simulink model "kalman_vision"  (R2013a)
settings: Solver=ode3  StartTime=0.0  StopTime=Inf  FixedStep=1/30  RelTol=1e-3
undefined symbols (not defined in the file or in its folder): none, serial, strel, videoinput
libraries: visionsinks x3, instrumentlib x3, simulink x2, visionstatistics x1, imaqlib x1, visiontextngfix x1, dspadpt3 x1, visionmorphops x1
settings Model: Creator=Michael  LastModifiedBy=nano

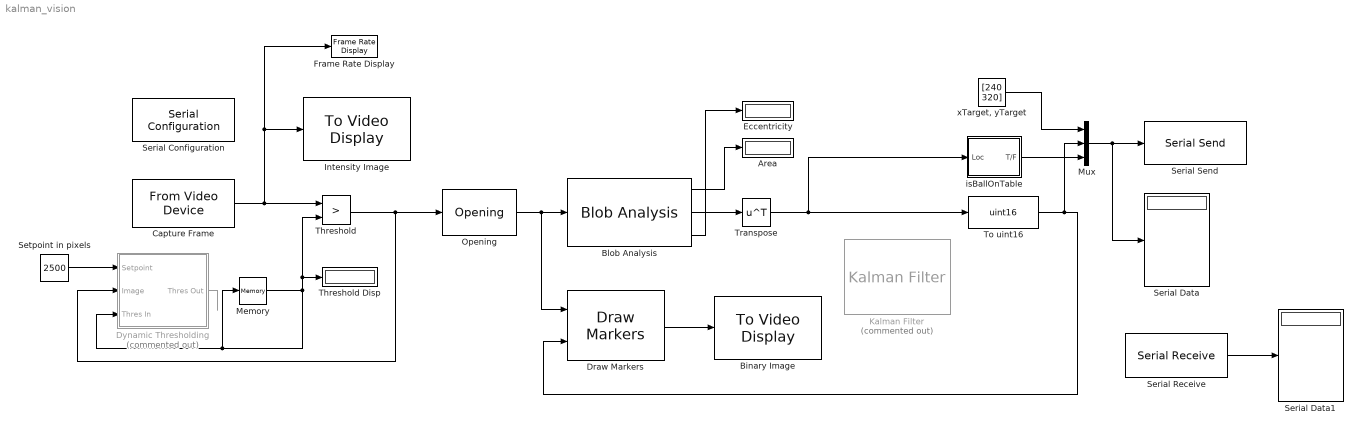
== system kalman_vision ==
  Area : Display
  Binary Image : visionsinks/To Video Display  inputType=Obsolete  imagePorts=One multidimensional signal  OutputDevice=On-screen video monitor  fullScreen=off  videoWindowX=-732  videoWindowY=343  saveWindowSize=off  videoWindowWidth=640  videoWindowHeight=480  dataOrg=Column-major  openAtMdlStart=on  isWindowOpen=off  inputColorFormat=RGB
  Blob Analysis : visionstatistics/Blob Analysis  Tag=vipblks_row_conv  area=on  centroid=on  bBox=off  majorAxis=off  minorAxis=off  angle=off  eccentricity=on  equivDiameterSq=off  extent=off  perimeter=off  maxBlobs=1  warnIfNumBlobsExceeded=off  isCount=off  useMinArea=on  minArea=700  useMaxArea=on  maxArea=2000  excludeBorderBlob=on  outDT=double  isOutVarDim=off  isFill=on  fillValues=-1  conn=8  isLabel=off  outputMode=Binary point scaling  outputWordLength=32  outputFracLength=16  firstCoeffMode=Binary point scaling  firstCoeffWordLength=16  firstCoeffFracLength=14  secondCoeffMode=Binary point scaling  secondCoeffWordLength=32  secondCoeffFracLength=16  accumMode=Binary point scaling  accumWordLength=32  accumFracLength=0  prodOutputMode=Binary point scaling  prodOutputWordLength=32  prodOutputFracLength=16  roundingMode=Floor  overflowMode=off
  Capture Frame : imaqlib/From Video Device  DeviceMenu=winvideo 1 (HP Prem AF Webcam KQ245AA)  Device=winvideo 1 (HP Prem AF Webcam KQ245AA)  ObjConstructor=videoinput('winvideo', 1)  VideoFormatMenu=MJPG_640x480  VideoFormat=MJPG_640x480  VideoSource=input1  ROIPosition=[0 0 480 640]  EnableHWTrigger=off  TriggerConfiguration=none/none  SampleTime=1/30  OutputPortsMode=One multidimensional signal  DataType=uint8  CanDoHWTrigger=no  ReturnedColorSpace=grayscale  BlockHandle=1913.0001  ROIWidth=640  ROIHeight=480  ROIColumn=0  ROIRow=0  EngXMLPath=C:\Program Files\MATLAB\R2013a\toolbox\imaq\imaq\private  DevXMLPath=C:\Program Files\MATLAB\R2013a\toolbox\imaq\imaqadaptors\win64  EngLibPath=C:\Program Files\MATLAB\R2013a\toolbox\imaq\imaqblks\imaqmex\win64  ColorSpace=grayscale  BayerSensorAlignment=grbg
  Draw Markers : visiontextngfix/Draw Markers  shape=Plus  size=40  fill=off  fillClrSource=Specify via dialog  display=White  intensity=200  color=[255 0 0]  opacity=0.6  viewport=Entire image  antialiasing=off  inType=Obsolete  imagePorts=One multidimensional signal  prodOutputMode=Binary point scaling  prodOutputWordLength=32  prodOutputFracLength=14  memoryMode=Specify word length  memoryWordLength=16  memoryFracLength=15  roundingMode=Floor  overflowMode=off
  Dynamic Thresholding : Subsystem  Commented=on
  Eccentricity : Display
  Frame Rate Display : visionsinks/Frame Rate Display  UpdateRate=30
  Intensity Image : visionsinks/To Video Display  inputType=Obsolete  imagePorts=One multidimensional signal  OutputDevice=On-screen video monitor  fullScreen=off  videoWindowX=-1279  videoWindowY=60  saveWindowSize=off  videoWindowWidth=640  videoWindowHeight=480  dataOrg=Column-major  openAtMdlStart=on  isWindowOpen=off  inputColorFormat=RGB
  Kalman Filter : dspadpt3/Kalman Filter  Commented=on  num_targets=1  sourceEnable=Always  isReset=on  X=[1; 1; 0; 0; 0; 0]  P=0.5*eye(6)  A=[1 0 1/30 0 (1/30^2)/2 0; 0 1 0 1/30 0 (1/30^2)/2; 0 0 1 0 1/30 0; 0 0 0 1 0 1/30; 0 0 0 0 1 0; 0 0 0 0 0 1]  sourceMeasure=Specify via Dialog  H=[1 0 0 0 0 0; 0 1 0 0 0 0]  Q=diag([(1/30^4)/4 (1/30^4)/4 (1/30)^2 (1/30)^2 1 1])  R=eye(2)  isOutputEstMeasure=on  isOutputEstState=off  isOutputEstError=off  isOutputPrdMeasure=off  isOutputPrdState=off  isOutputPrdError=off
  Memory : Memory  X0=200  InheritSampleTime=on
  Mux : Mux  Inputs=3
  Opening : visionmorphops/Opening  nhoodsrc=Specify via dialog  strel=strel('disk',7)
  Serial Configuration : instrumentlib/Serial Configuration  Priority=-200000  ComPortMenu=COM7  ComPort=COM7  ObjConstructor=serial('COM7');  BaudRate=115200  DataBits=8  Parity=none  StopBits=1  FlowControl=none  Timeout=10  ByteOrder=LittleEndian
  Serial Data : Display
  Serial Data1 : Display
  Serial Receive : instrumentlib/Serial Receive  ComPortMenu=COM7  ComPort=COM7  ObjConstructor=serial('COM7');  Terminator=<none>  DataSize="[5  1]"  DataType=uint16  EnableBlockingMode=on  ActionDataUnavailable=Output custom value  CustomValue=0  SampleTime=1/30
  Serial Send : instrumentlib/Serial Send  ComPortMenu=COM7  ComPort=COM7  ObjConstructor=serial('COM7');  Terminator=<none>  EnableBlockingMode=off
  Setpoint in pixels : Constant  Value=2500  OutDataTypeStr=uint16
  Threshold : RelationalOperator  Operator=>  OutDataTypeStr=boolean  ZeroCross=off
  Threshold Disp : Display
  To uint16 : DataTypeConversion  OutDataTypeStr=uint16
  Transpose : Math  Operator=transpose  SaturateOnIntegerOverflow=on
  isBallOnTable : Subsystem
  "xTarget, yTarget" : Constant  Value=[240 320]  OutDataTypeStr=uint16
  wires:
  Capture Frame/1 -> Frame Rate Display/1, Intensity Image/1, Threshold/1
  To uint16/1 -> Mux/2, Draw Markers/2
  Blob Analysis/1 -> Area/1
  Opening/1 -> Draw Markers/1, Blob Analysis/1
  Draw Markers/1 -> Binary Image/1
  Blob Analysis/3 -> Eccentricity/1
  Blob Analysis/2 -> Transpose/1
  Transpose/1 -> isBallOnTable/1(Loc), To uint16/1
  Mux/1 -> Serial Send/1, Serial Data/1
  "xTarget, yTarget"/1 -> Mux/1
  isBallOnTable/1(T/F) -> Mux/3
  Threshold/1 -> Dynamic Thresholding/2(Image), Opening/1
  Dynamic Thresholding/1(Thres Out) -> ?
  Setpoint in pixels/1 -> Dynamic Thresholding/1(Setpoint)
  Memory/1 -> Threshold/2, Threshold Disp/1, Memory/1, Dynamic Thresholding/3(Thres In)
  Serial Receive/1 -> Serial Data1/1

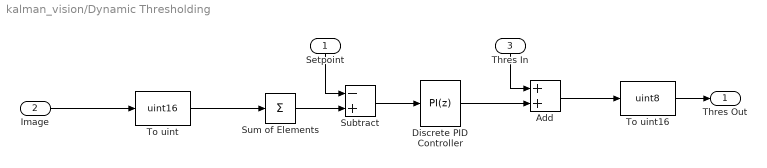
== system kalman_vision/Dynamic Thresholding ==
  Setpoint : Inport
  Image : Inport  Port=2
  Thres In : Inport  Port=3
  Add : Sum
  Discrete PID Controller : simulink/Continuous/PID Controller  Controller=PI  TimeDomain=Discrete-time  SampleTime=-1  IntegratorMethod=Forward Euler  FilterMethod=Forward Euler  Form=Parallel  P=1/5000  I=1/5000  D=0  N=100  InitialConditionSource=internal  InitialConditionForIntegrator=0  InitialConditionForFilter=0  ExternalReset=none  LimitOutput=off  UpperSaturationLimit=50  LowerSaturationLimit=-50  LinearizeAsGain=off  AntiWindupMode=none  Kb=1  TrackingMode=off  Kt=1  PParamMin=[]  PParamMax=[]  IParamMin=[]  IParamMax=[]  DParamMin=[]  DParamMax=[]  NParamMin=[]  NParamMax=[]  KbParamMin=[]  KbParamMax=[]  KtParamMin=[]  KtParamMax=[]  POutMin=[]  POutMax=[]  IOutMin=[]  IOutMax=[]  DOutMin=[]  DOutMax=[]  NOutMin=[]  NOutMax=[]  KbOutMin=[]  KbOutMax=[]  KtOutMin=[]  KtOutMax=[]  IntegratorOutMin=[]  IntegratorOutMax=[]  FilterOutMin=[]  FilterOutMax=[]  SumOutMin=[]  SumOutMax=[]  SumI1OutMin=[]  SumI1OutMax=[]  SumI2OutMin=[]  SumI2OutMax=[]  SumI3OutMin=[]  SumI3OutMax=[]  SumDOutMin=[]  SumDOutMax=[]  SaturationOutMin=[]  SaturationOutMax=[]  IntegratorContinuousStateAttributes=''  IntegratorStateMustResolveToSignalObject=off  IntegratorRTWStateStorageClass=Auto  FilterContinuousStateAttributes=''  FilterStateMustResolveToSignalObject=off  FilterRTWStateStorageClass=Auto
  Subtract : Sum  Inputs=-+  AccumDataTypeStr=single
  Sum of Elements : Sum  Inputs=+
  To uint : DataTypeConversion  OutDataTypeStr=uint16
  To uint16 : DataTypeConversion  OutDataTypeStr=uint8
  Thres Out : Outport
  wires:
  Sum of Elements/1 -> Subtract/2
  Discrete PID Controller/1 -> Add/2
  Subtract/1 -> Discrete PID Controller/1
  Setpoint/1 -> Subtract/1
  Add/1 -> To uint16/1
  Thres In/1 -> Add/1
  Image/1 -> To uint/1
  To uint/1 -> Sum of Elements/1
  To uint16/1 -> Thres Out/1

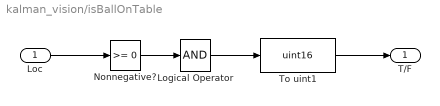
== system kalman_vision/isBallOnTable ==
  Loc : Inport
  Logical Operator : Logic  Inputs=1  AllPortsSameDT=off  OutDataTypeStr=boolean
  Nonnegative? : simulink/Logic and Bit Operations/Compare To Zero  relop=>=  OutDataTypeStr=boolean  ZeroCross=off
  To uint1 : DataTypeConversion  OutDataTypeStr=uint16
  T/F : Outport
  wires:
  Logical Operator/1 -> To uint1/1
  Nonnegative?/1 -> Logical Operator/1
  To uint1/1 -> T/F/1
  Loc/1 -> Nonnegative?/1
